simulink model "TiltCopter_TOSTO_v3"  (R2015a)
settings: Solver=ode45  StartTime=0.0  StopTime=10  RelTol=1e-3
values from neighbouring files (symbols this model uses):
  b = 0.55/2    (= 0.275)    [TiltCopter_Parameters_TOSTO_v3.m]
  B0 = 1.399e04    (= 13990)    [TiltCopter_Parameters_TOSTO_v3.m]
  B1 = 1150    [TiltCopter_Parameters_TOSTO_v3.m]
  B2 = 37.46    [TiltCopter_Parameters_TOSTO_v3.m]
  B3 = 1    [TiltCopter_Parameters_TOSTO_v3.m]
  degtorad = pi/180    (= 0.0174532925199)    [TiltCopter_Parameters_TOSTO_v3.m]
  dLMN = [dLdp  0    0 ... (first row only)    [TiltCopter_Parameters_TOSTO_v3.m]
  g = 9.81    [TiltCopter_Parameters_TOSTO_v3.m]
  I_Pi = diag([8.450e-5 8.450e-5 4.580e-5])    [TiltCopter_Parameters_TOSTO_v3.m]
  In = diag([Ixx Iyy Izz])    [TiltCopter_Parameters_TOSTO_v3.m]
  InInv = In\eye(3)    [TiltCopter_Parameters_TOSTO_v3.m]
  KaD = 5.4    [TiltCopter_Parameters_TOSTO_v3.m]
  KaI = 3.6    [TiltCopter_Parameters_TOSTO_v3.m]
  KaN = 38    [TiltCopter_Parameters_TOSTO_v3.m]
  KaP = 8.0    (= 8)    [TiltCopter_Parameters_TOSTO_v3.m]
  Kba = sqrt(KaD/KaI)    [TiltCopter_Parameters_TOSTO_v3.m]
  Kbp = sqrt(Kdp/Kip)    [TiltCopter_Parameters_TOSTO_v3.m]
  Kbq = sqrt(Kdq/Kiq)    [TiltCopter_Parameters_TOSTO_v3.m]
  Kbr = sqrt(Kdr/Kir)    [TiltCopter_Parameters_TOSTO_v3.m]
  Kdp = 0.0499    [TiltCopter_Parameters_TOSTO_v3.m]
  Kdq = 0.0499    [TiltCopter_Parameters_TOSTO_v3.m]
  Kdr = 0.0153    [TiltCopter_Parameters_TOSTO_v3.m]
  Kip = 0.304    [TiltCopter_Parameters_TOSTO_v3.m]
  Kiq = 0.304    [TiltCopter_Parameters_TOSTO_v3.m]
  Kir = 0.125    [TiltCopter_Parameters_TOSTO_v3.m]
  KPD = 0.00512    [TiltCopter_Parameters_TOSTO_v3.m]
  KPP = 1.61    [TiltCopter_Parameters_TOSTO_v3.m]
  Kpp = 0.298    [TiltCopter_Parameters_TOSTO_v3.m]
  Kpq = 0.298    [TiltCopter_Parameters_TOSTO_v3.m]
  Kpr = 0.135    [TiltCopter_Parameters_TOSTO_v3.m]
  Kq = Cq*ro*A*R^3    (= 2.88925724261e-07)    [TiltCopter_Parameters_TOSTO_v3.m]
  KRD = 0.00512    [TiltCopter_Parameters_TOSTO_v3.m]
  KRP = 1.61    [TiltCopter_Parameters_TOSTO_v3.m]
  Kt = Ct*ro*A*R^2    (= 2.46191978476e-05)    [TiltCopter_Parameters_TOSTO_v3.m]
  m = 1.510    (= 1.51)    [TiltCopter_Parameters_TOSTO_v3.m]
  m_servo = p(1)    [TiltCopter_Parameters_TOSTO_v3.m]
  Mb = diag([m m m])    [TiltCopter_Parameters_TOSTO_v3.m]
  MbInv = Mb\eye(3)    [TiltCopter_Parameters_TOSTO_v3.m]
  N = 1/Tf    (= 100)    [TiltCopter_Parameters_TOSTO_v3.m]
  omega_hover = OMEhov    [TiltCopter_Parameters_TOSTO_v3.m]
  pitchMax = pi/6    (= 0.523598775598)    [TiltCopter_Parameters_TOSTO_v3.m]
  q_servo = p(2)    [TiltCopter_Parameters_TOSTO_v3.m]
  rollMax = pi/6    (= 0.523598775598)    [TiltCopter_Parameters_TOSTO_v3.m]
  satp = 1.5    [TiltCopter_Parameters_TOSTO_v3.m]
  satq = 1.5    [TiltCopter_Parameters_TOSTO_v3.m]
  satr = 1    [TiltCopter_Parameters_TOSTO_v3.m]
  ServoMotor_Gain = 1.409e04    (= 14090)    [TiltCopter_Parameters_TOSTO_v3.m]
  tau = 0.055257    [TiltCopter_Parameters_TOSTO_v3.m]
  U = [-1; 0; 0; 0]    [Main_tiltCopter_TOSTO_v3.m]
  x1 = [m q]    [TiltCopter_Parameters_TOSTO_v3.m]
  yawRateMax = pi/2    (= 1.57079632679)    [TiltCopter_Parameters_TOSTO_v3.m]
undefined symbols (not defined in the file or in its folder): i, KPI, KRI
libraries: aerolibutil x10, simulink x6
(part 1 of 2)
settings Model: PauseTimes=2  Creator=Claudio  LastModifiedBy=Claudio

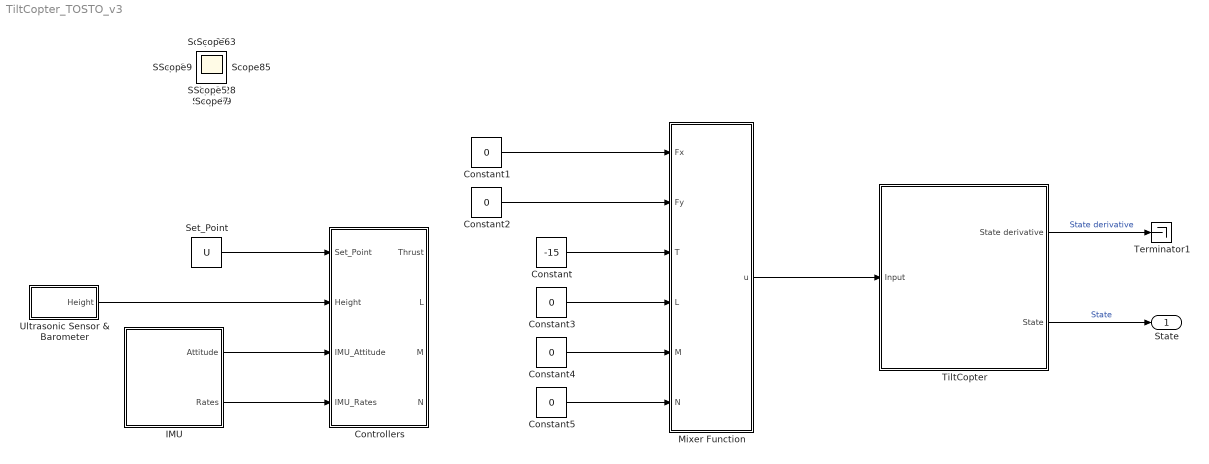
== system TiltCopter_TOSTO_v3 ==
  Constant : Constant  Value=-15
  Constant{1..5} (5 alike) : Constant  Value=0
  Controllers : Subsystem
  IMU : Subsystem
  Mixer Function : Subsystem
  Set_Point : Constant  Value=U
  Terminator1 : Terminator
  TiltCopter : Subsystem
      mask Display:
      | % image(imread(''))
      | port_label('input',1,'u')
      | port_label('output',1,'Xdot')
      | port_label('output',2,'X')
  Ultrasonic Sensor & Barometer : Subsystem
  State : Outport
  Scope{,1..29} (30 alike) : Scope
      Scope settings: SaveName=ScopeData2
      Scope1 settings: SaveName=ScopeData3
      Scope10 settings: SaveName=ScopeData14
      Scope11 settings: SaveName=ScopeData15
      Scope12 settings: SaveName=ScopeData16
      Scope13 settings: SaveName=ScopeData17
      Scope14 settings: SaveName=ScopeData18
      Scope15 settings: SaveName=ScopeData19
      Scope16 settings: SaveName=ScopeData20
      Scope17 settings: SaveName=ScopeData21
      Scope18 settings: SaveName=ScopeData22
      Scope19 settings: SaveName=ScopeData23
      Scope2 settings: SaveName=ScopeData4
      Scope20 settings: SaveName=ScopeData24
      Scope21 settings: SaveName=ScopeData25
      Scope22 settings: SaveName=ScopeData26
      Scope23 settings: SaveName=ScopeData27
      Scope24 settings: SaveName=ScopeData28
      Scope25 settings: SaveName=ScopeData31
      Scope26 settings: SaveName=ScopeData30
      Scope27 settings: ShowLegends=on  SaveName=ScopeData32
      Scope28 settings: SaveName=ScopeData33
      Scope29 settings: SaveName=ScopeData34
      Scope3 settings: SaveName=ScopeData5
      Scope4 settings: SaveName=ScopeData8
      Scope5 settings: TimeRange=20  SaveName=ScopeData9
      Scope6 settings: SaveName=ScopeData10
      Scope7 settings: SaveName=ScopeData11
      Scope8 settings: SaveName=ScopeData12
      Scope9 settings: SaveName=ScopeData13
  wires:
  TiltCopter/2(State) -> State/1  "State"
  TiltCopter/1(State derivative) -> Terminator1/1  "State derivative"
  Constant1/1 -> Mixer Function/1(Fx)
  Constant2/1 -> Mixer Function/2(Fy)
  Mixer Function/1(u) -> TiltCopter/1(Input)
  Set_Point/1 -> Controllers/1(Set_Point)
  IMU/1(Attitude) -> Controllers/3(IMU_Attitude)
  IMU/2(Rates) -> Controllers/4(IMU_Rates)
  Ultrasonic Sensor & Barometer/1(Height) -> Controllers/2(Height)
  Constant/1 -> Mixer Function/3(T)
  Constant5/1 -> Mixer Function/6(N)
  Constant4/1 -> Mixer Function/5(M)
  Constant3/1 -> Mixer Function/4(L)

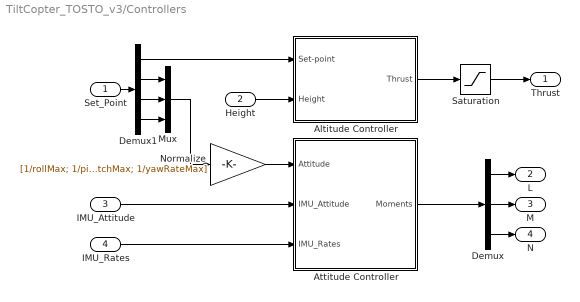
== system TiltCopter_TOSTO_v3/Controllers ==
  Set_Point : Inport
  Height : Inport  Port=2
  IMU_Attitude : Inport  Port=3
  IMU_Rates : Inport  Port=4
  Altitude Controller : Subsystem
  Attitude Controller : Subsystem
  Demux : Demux  Outputs=3
  Demux1 : Demux
  Mux : Mux  Inputs=3
  Normalize : Gain  Gain=[1/rollMax; 1/pitchMax; 1/yawRateMax]
  Saturation : Saturate  UpperLimit=0  LowerLimit=-80
  Thrust : Outport
  L : Outport  Port=2
  M : Outport  Port=3
  N : Outport  Port=4
  wires:
  IMU_Rates/1 -> Attitude Controller/3(IMU_Rates)
  Demux/1 -> L/1
  Demux/2 -> M/1
  Demux/3 -> N/1
  Set_Point/1 -> Demux1/1
  Demux1/3 -> Mux/2
  Demux1/4 -> Mux/3
  IMU_Attitude/1 -> Attitude Controller/2(IMU_Attitude)
  Mux/1 -> Normalize/1
  Normalize/1 -> Attitude Controller/1(Attitude)
  Demux1/1 -> Altitude Controller/1(Set-point)
  Height/1 -> Altitude Controller/2(Height)
  Altitude Controller/1(Thrust) -> Saturation/1
  Saturation/1 -> Thrust/1
  Attitude Controller/1(Moments) -> Demux/1
  Demux1/2 -> Mux/1

== system TiltCopter_TOSTO_v3/IMU ==
  Attitude : Outport
  Rates : Outport  Port=2
  wires:
  [Omega_b] -> Rates/1
  [Alpha_e] -> Attitude/1

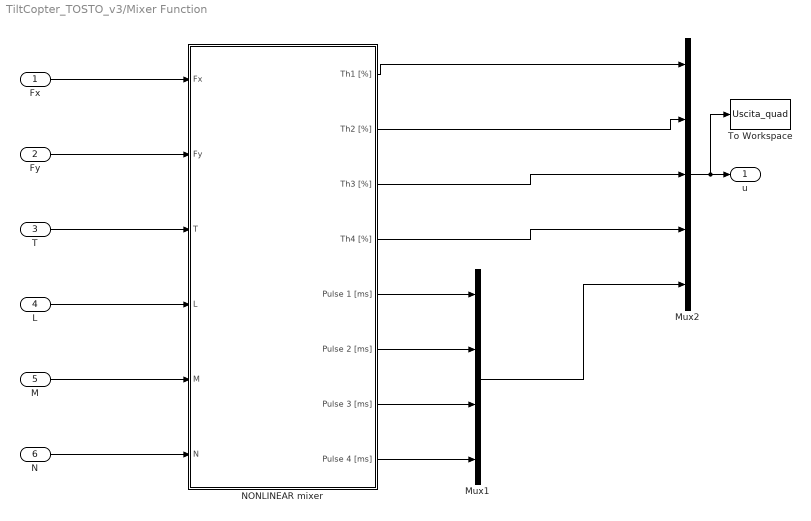
== system TiltCopter_TOSTO_v3/Mixer Function ==
  Fx : Inport
  Fy : Inport  Port=2
  T : Inport  Port=3
  L : Inport  Port=4
  M : Inport  Port=5
  N : Inport  Port=6
  Mux1 : Mux
  Mux2 : Mux  Inputs=5
  NONLINEAR mixer : Subsystem
  To Workspace : ToWorkspace  VariableName=Uscita_quad  SaveFormat=Timeseries  SampleTime=-1
  u : Outport
  wires:
  Mux2/1 -> To Workspace/1, u/1
  Fy/1 -> NONLINEAR mixer/2(Fy)
  Fx/1 -> NONLINEAR mixer/1(Fx)
  T/1 -> NONLINEAR mixer/3(T)
  L/1 -> NONLINEAR mixer/4(L)
  N/1 -> NONLINEAR mixer/6(N)
  M/1 -> NONLINEAR mixer/5(M)
  Mux1/1 -> Mux2/5
  NONLINEAR mixer/5(Pulse 1 [ms]) -> Mux1/1
  NONLINEAR mixer/6(Pulse 2 [ms]) -> Mux1/2
  NONLINEAR mixer/7(Pulse 3 [ms]) -> Mux1/3
  NONLINEAR mixer/8(Pulse 4 [ms]) -> Mux1/4
  NONLINEAR mixer/4(Th4 [%]) -> Mux2/4
  NONLINEAR mixer/3(Th3 [%]) -> Mux2/3
  NONLINEAR mixer/2(Th2 [%]) -> Mux2/2
  NONLINEAR mixer/1(Th1 [%]) -> Mux2/1

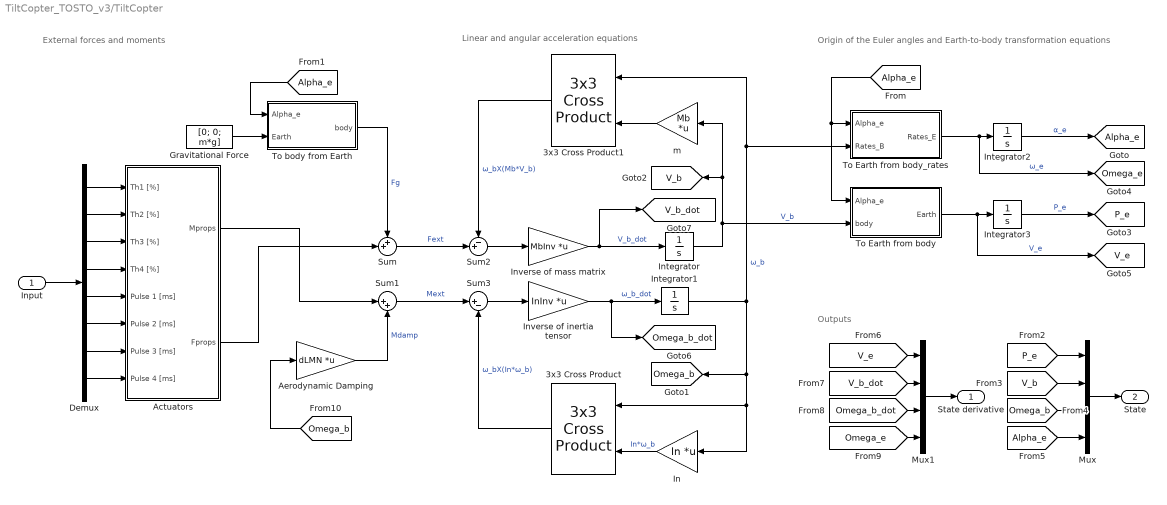
== system TiltCopter_TOSTO_v3/TiltCopter ==
  note: External forces and moments
  note: Outputs
  note: Origin of the Euler angles and Earth-to-body transformation equations
  note: Linear and angular acceleration equations
  Input : Inport
  3x3 Cross Product : aerolibutil/3x3 Cross Product
  3x3 Cross Product1 : aerolibutil/3x3 Cross Product
  Actuators : Subsystem
  Aerodynamic Damping : Gain  Gain=dLMN  Multiplication=Matrix(K*u)
  Demux : Demux  Outputs=8
  Gravitational Force : Constant  Value=[0; 0; m*g]
  In : Gain  Gain=In  Multiplication=Matrix(K*u)
  Integrator : Integrator  InitialCondition=[0; 0; 0]  UpperSaturationLimit=20
  Integrator1 : Integrator  InitialCondition=[0; 0; 0]
  Integrator2 : Integrator  InitialCondition=[0; 0; 0]
  Integrator3 : Integrator  InitialCondition=[0; 0; 0]
  Inverse of inertia tensor : Gain  Gain=InInv  Multiplication=Matrix(K*u)
  Inverse of mass matrix : Gain  Gain=MbInv  Multiplication=Matrix(K*u)
  Mux : Mux
  Mux1 : Mux
  Sum : Sum  Inputs=++|
  Sum1 : Sum  Inputs=|++
  Sum2 : Sum  Inputs=-+|
  Sum3 : Sum  Inputs=|+-
  To Earth from body : MATLAB Function  TreatAsAtomicUnit=on
  To Earth from body_rates : MATLAB Function  TreatAsAtomicUnit=on
  To body from Earth : MATLAB Function  TreatAsAtomicUnit=on
  m : Gain  Gain=Mb  Multiplication=Matrix(K*u)
  State derivative : Outport
  State : Outport  Port=2
  tag scope: Alpha_e=global, Omega_b=global, Omega_b_dot=global, Omega_e=global, P_e=global, V_b=global, V_b_dot=global, V_e=global
  wires:
  To Earth from body_rates/1(Rates_E) -> Integrator2/1, [Omega_e]  "ω_e"
  [P_e] -> Mux/1
  3x3 Cross Product/1 -> Sum3/2  "ω_bX(In*ω_b)"
  [V_b_dot] -> Mux1/2
  Mux/1 -> State/1
  Mux1/1 -> State derivative/1
  [V_b] -> Mux/2
  [Alpha_e] -> Mux/4
  [Omega_b] -> Mux/3
  Demux/4 -> Actuators/4(Th4 [%])
  [Omega_e] -> Mux1/4
  [Omega_b_dot] -> Mux1/3
  [V_e] -> Mux1/1
  Demux/3 -> Actuators/3(Th3 [%])
  Inverse of mass matrix/1 -> Integrator/1, [V_b_dot]  "V_b_dot"
  Integrator/1 -> To Earth from body/2(body), m/1, [V_b]  "V_b"
  [Alpha_e] -> To Earth from body/1(Alpha_e), To Earth from body_rates/1(Alpha_e)
  Integrator1/1 -> To Earth from body_rates/2(Rates_B), 3x3 Cross Product1/1, 3x3 Cross Product/1, In/1, [Omega_b]  "ω_b"
  Sum3/1 -> Inverse of inertia tensor/1
  Sum2/1 -> Inverse of mass matrix/1
  m/1 -> 3x3 Cross Product1/2
  Sum/1 -> Sum2/2  "Fext"
  Sum1/1 -> Sum3/1  "Mext"
  Demux/1 -> Actuators/1(Th1 [%])
  Demux/2 -> Actuators/2(Th2 [%])
  Inverse of inertia tensor/1 -> Integrator1/1, [Omega_b_dot]  "ω_b_dot"
  3x3 Cross Product1/1 -> Sum2/1  "ω_bX(Mb*V_b)"
  Integrator2/1 -> [Alpha_e]  "α_e"
  Aerodynamic Damping/1 -> Sum1/2  "Mdamp"
  Integrator3/1 -> [P_e]  "P_e"
  In/1 -> 3x3 Cross Product/2  "In*ω_b"
  [Omega_b] -> Aerodynamic Damping/1
  To Earth from body/1(Earth) -> [V_e], Integrator3/1  "V_e"
  To body from Earth/1(body) -> Sum/1  "Fg"
  Gravitational Force/1 -> To body from Earth/2(Earth)
  [Alpha_e] -> To body from Earth/1(Alpha_e)
  Input/1 -> Demux/1
  Demux/5 -> Actuators/5(Pulse 1 [ms])
  Demux/6 -> Actuators/6(Pulse 2 [ms])
  Demux/7 -> Actuators/7(Pulse 3 [ms])
  Demux/8 -> Actuators/8(Pulse 4 [ms])
  Actuators/1(Mprops) -> Sum1/1
  Actuators/2(Fprops) -> Sum/2

== system TiltCopter_TOSTO_v3/Ultrasonic Sensor & Barometer ==
  Bias_u : Bias
  Demux : Demux  Outputs=3
  Sum : Sum  Inputs=|++
  Terminator1 : Terminator
  Terminator2 : Terminator
  White Noise_u : RandomNumber  DisableCoverage=on  Variance=0*0.00001  SampleTime=0.01
  Height : Outport
  wires:
  Sum/1 -> Height/1
  Demux/2 -> Terminator1/1  "E"
  [P_e] -> Demux/1
  Bias_u/1 -> Sum/1
  White Noise_u/1 -> Sum/2
  Demux/3 -> Bias_u/1  "D"
  Demux/1 -> Terminator2/1  "N"

== system TiltCopter_TOSTO_v3/Controllers/Altitude Controller ==
  Set-point : Inport
  Height : Inport  Port=2
  Constant : Constant  Value=m*g
  Normalize : Gain
  PD Controller : simulink/Continuous/PID Controller  Controller=PID  TimeDomain=Continuous-time  SampleTime=-1  IntegratorMethod=Forward Euler  FilterMethod=Trapezoidal  Form=Parallel  UseFilter=on  ControllerParametersSource=internal  P=KaP  I=KaI  D=KaD  N=KaN  InitialConditionSource=internal  InitialConditionForIntegrator=0  InitialConditionForFilter=0  ExternalReset=none  LimitOutput=on  UpperSaturationLimit=10  LowerSaturationLimit=-10  LinearizeAsGain=on  AntiWindupMode=back-calculation  Kb=Kba  TrackingMode=off  Kt=1  PParamMin=[]  PParamMax=[]  IParamMin=[]  IParamMax=[]  DParamMin=[]  DParamMax=[]  NParamMin=[]  NParamMax=[]  KbParamMin=[]  KbParamMax=[]  KtParamMin=[]  KtParamMax=[]  POutMin=[]  POutMax=[]  IOutMin=[]  IOutMax=[]  DOutMin=[]  DOutMax=[]  NOutMin=[]  NOutMax=[]  KbOutMin=[]  KbOutMax=[]  KtOutMin=[]  KtOutMax=[]  IntegratorOutMin=[]  IntegratorOutMax=[]  FilterOutMin=[]  FilterOutMax=[]  SumOutMin=[]  SumOutMax=[]  SumI1OutMin=[]  SumI1OutMax=[]  SumI2OutMin=[]  SumI2OutMax=[]  SumI3OutMin=[]  SumI3OutMax=[]  SumDOutMin=[]  SumDOutMax=[]  SaturationOutMin=[]  SaturationOutMax=[]  IntegratorContinuousStateAttributes=''  IntegratorStateMustResolveToSignalObject=off  IntegratorRTWStateStorageClass=Auto  FilterContinuousStateAttributes=''  FilterStateMustResolveToSignalObject=off  FilterRTWStateStorageClass=Auto  DifferentiatorICPrevScaledInput=0  DifferentiatorOutMin=[]  DifferentiatorOutMax=[]
  Sum1 : Sum  Inputs=-+|
  Sum2 : Sum  Inputs=|+-
  Thrust : Outport
  wires:
  Sum2/1 -> PD Controller/1
  Height/1 -> Sum2/2
  Sum1/1 -> Thrust/1
  Constant/1 -> Sum1/1
  Set-point/1 -> Sum2/1
  PD Controller/1 -> Normalize/1
  Normalize/1 -> Sum1/2

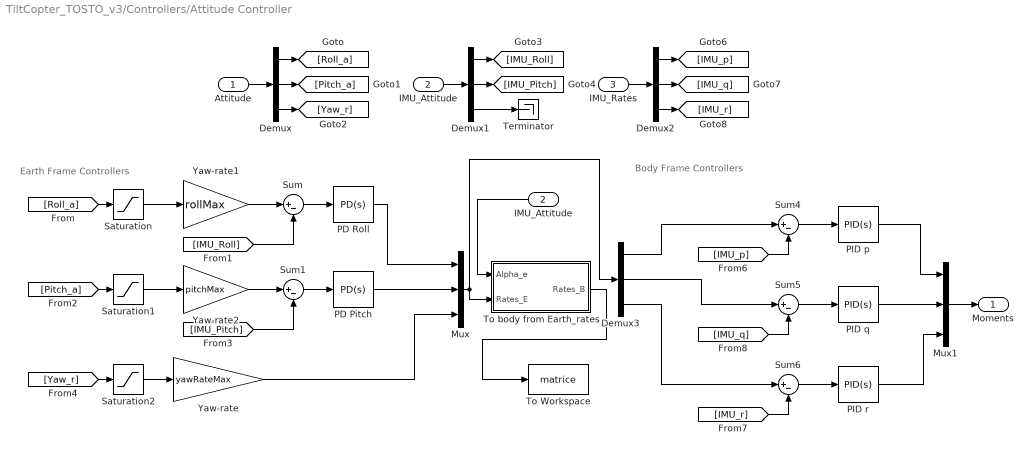
== system TiltCopter_TOSTO_v3/Controllers/Attitude Controller ==
  note: Body Frame Controllers
  note: Earth Frame Controllers
  Attitude : Inport
  IMU_Attitude : Inport  Port=2
  IMU_Rates : Inport  Port=3
  Demux{,1..3} (4 alike) : Demux  Outputs=3
  "IMU_Attitude " : InportShadow  Port=2
  Mux : Mux  Inputs=3
  Mux1 : Mux  Inputs=3
  PD Pitch : simulink/Continuous/PID Controller  Controller=PD  TimeDomain=Continuous-time  SampleTime=-1  IntegratorMethod=Forward Euler  FilterMethod=Forward Euler  Form=Parallel  UseFilter=on  ControllerParametersSource=internal  P=KPP  I=KPI  D=KPD  N=N  InitialConditionSource=internal  InitialConditionForIntegrator=0  InitialConditionForFilter=0  ExternalReset=none  LimitOutput=off  UpperSaturationLimit=inf  LowerSaturationLimit=-inf  LinearizeAsGain=on  AntiWindupMode=none  Kb=1  TrackingMode=off  Kt=1  PParamMin=[]  PParamMax=[]  IParamMin=[]  IParamMax=[]  DParamMin=[]  DParamMax=[]  NParamMin=[]  NParamMax=[]  KbParamMin=[]  KbParamMax=[]  KtParamMin=[]  KtParamMax=[]  POutMin=[]  POutMax=[]  IOutMin=[]  IOutMax=[]  DOutMin=[]  DOutMax=[]  NOutMin=[]  NOutMax=[]  KbOutMin=[]  KbOutMax=[]  KtOutMin=[]  KtOutMax=[]  IntegratorOutMin=[]  IntegratorOutMax=[]  FilterOutMin=[]  FilterOutMax=[]  SumOutMin=[]  SumOutMax=[]  SumI1OutMin=[]  SumI1OutMax=[]  SumI2OutMin=[]  SumI2OutMax=[]  SumI3OutMin=[]  SumI3OutMax=[]  SumDOutMin=[]  SumDOutMax=[]  SaturationOutMin=[]  SaturationOutMax=[]  IntegratorContinuousStateAttributes=''  IntegratorStateMustResolveToSignalObject=off  IntegratorRTWStateStorageClass=Auto  FilterContinuousStateAttributes=''  FilterStateMustResolveToSignalObject=off  FilterRTWStateStorageClass=Auto  DifferentiatorICPrevScaledInput=0  DifferentiatorOutMin=[]  DifferentiatorOutMax=[]
  PD Roll : simulink/Continuous/PID Controller  Controller=PD  TimeDomain=Continuous-time  SampleTime=-1  IntegratorMethod=Forward Euler  FilterMethod=Forward Euler  Form=Parallel  UseFilter=on  ControllerParametersSource=internal  P=KRP  I=KRI  D=KRD  N=N  InitialConditionSource=internal  InitialConditionForIntegrator=0  InitialConditionForFilter=0  ExternalReset=none  LimitOutput=off  UpperSaturationLimit=inf  LowerSaturationLimit=-inf  LinearizeAsGain=on  AntiWindupMode=none  Kb=1  TrackingMode=off  Kt=1  PParamMin=[]  PParamMax=[]  IParamMin=[]  IParamMax=[]  DParamMin=[]  DParamMax=[]  NParamMin=[]  NParamMax=[]  KbParamMin=[]  KbParamMax=[]  KtParamMin=[]  KtParamMax=[]  POutMin=[]  POutMax=[]  IOutMin=[]  IOutMax=[]  DOutMin=[]  DOutMax=[]  NOutMin=[]  NOutMax=[]  KbOutMin=[]  KbOutMax=[]  KtOutMin=[]  KtOutMax=[]  IntegratorOutMin=[]  IntegratorOutMax=[]  FilterOutMin=[]  FilterOutMax=[]  SumOutMin=[]  SumOutMax=[]  SumI1OutMin=[]  SumI1OutMax=[]  SumI2OutMin=[]  SumI2OutMax=[]  SumI3OutMin=[]  SumI3OutMax=[]  SumDOutMin=[]  SumDOutMax=[]  SaturationOutMin=[]  SaturationOutMax=[]  IntegratorContinuousStateAttributes=''  IntegratorStateMustResolveToSignalObject=off  IntegratorRTWStateStorageClass=Auto  FilterContinuousStateAttributes=''  FilterStateMustResolveToSignalObject=off  FilterRTWStateStorageClass=Auto  DifferentiatorICPrevScaledInput=0  DifferentiatorOutMin=[]  DifferentiatorOutMax=[]
  PID p : simulink/Continuous/PID Controller  Controller=PID  TimeDomain=Continuous-time  SampleTime=-1  IntegratorMethod=Forward Euler  FilterMethod=Forward Euler  Form=Parallel  UseFilter=on  ControllerParametersSource=internal  P=Kpp  I=Kip  D=Kdp  N=N  InitialConditionSource=internal  InitialConditionForIntegrator=0  InitialConditionForFilter=0  ExternalReset=none  LimitOutput=on  UpperSaturationLimit=satp  LowerSaturationLimit=-satp  LinearizeAsGain=on  AntiWindupMode=back-calculation  Kb=Kbp  TrackingMode=off  Kt=1  PParamMin=[]  PParamMax=[]  IParamMin=[]  IParamMax=[]  DParamMin=[]  DParamMax=[]  NParamMin=[]  NParamMax=[]  KbParamMin=[]  KbParamMax=[]  KtParamMin=[]  KtParamMax=[]  POutMin=[]  POutMax=[]  IOutMin=[]  IOutMax=[]  DOutMin=[]  DOutMax=[]  NOutMin=[]  NOutMax=[]  KbOutMin=[]  KbOutMax=[]  KtOutMin=[]  KtOutMax=[]  IntegratorOutMin=[]  IntegratorOutMax=[]  FilterOutMin=[]  FilterOutMax=[]  SumOutMin=[]  SumOutMax=[]  SumI1OutMin=[]  SumI1OutMax=[]  SumI2OutMin=[]  SumI2OutMax=[]  SumI3OutMin=[]  SumI3OutMax=[]  SumDOutMin=[]  SumDOutMax=[]  SaturationOutMin=[]  SaturationOutMax=[]  IntegratorContinuousStateAttributes=''  IntegratorStateMustResolveToSignalObject=off  IntegratorRTWStateStorageClass=Auto  FilterContinuousStateAttributes=''  FilterStateMustResolveToSignalObject=off  FilterRTWStateStorageClass=Auto  DifferentiatorICPrevScaledInput=0  DifferentiatorOutMin=[]  DifferentiatorOutMax=[]
  PID q : simulink/Continuous/PID Controller  Controller=PID  TimeDomain=Continuous-time  SampleTime=-1  IntegratorMethod=Forward Euler  FilterMethod=Forward Euler  Form=Parallel  UseFilter=on  ControllerParametersSource=internal  P=Kpq  I=Kiq  D=Kdq  N=N  InitialConditionSource=internal  InitialConditionForIntegrator=0  InitialConditionForFilter=0  ExternalReset=none  LimitOutput=on  UpperSaturationLimit=satq  LowerSaturationLimit=-satq  LinearizeAsGain=on  AntiWindupMode=back-calculation  Kb=Kbq  TrackingMode=off  Kt=1  PParamMin=[]  PParamMax=[]  IParamMin=[]  IParamMax=[]  DParamMin=[]  DParamMax=[]  NParamMin=[]  NParamMax=[]  KbParamMin=[]  KbParamMax=[]  KtParamMin=[]  KtParamMax=[]  POutMin=[]  POutMax=[]  IOutMin=[]  IOutMax=[]  DOutMin=[]  DOutMax=[]  NOutMin=[]  NOutMax=[]  KbOutMin=[]  KbOutMax=[]  KtOutMin=[]  KtOutMax=[]  IntegratorOutMin=[]  IntegratorOutMax=[]  FilterOutMin=[]  FilterOutMax=[]  SumOutMin=[]  SumOutMax=[]  SumI1OutMin=[]  SumI1OutMax=[]  SumI2OutMin=[]  SumI2OutMax=[]  SumI3OutMin=[]  SumI3OutMax=[]  SumDOutMin=[]  SumDOutMax=[]  SaturationOutMin=[]  SaturationOutMax=[]  IntegratorContinuousStateAttributes=''  IntegratorStateMustResolveToSignalObject=off  IntegratorRTWStateStorageClass=Auto  FilterContinuousStateAttributes=''  FilterStateMustResolveToSignalObject=off  FilterRTWStateStorageClass=Auto  DifferentiatorICPrevScaledInput=0  DifferentiatorOutMin=[]  DifferentiatorOutMax=[]
  PID r : simulink/Continuous/PID Controller  Controller=PID  TimeDomain=Continuous-time  SampleTime=-1  IntegratorMethod=Forward Euler  FilterMethod=Forward Euler  Form=Parallel  UseFilter=on  ControllerParametersSource=internal  P=Kpr  I=Kir  D=Kdr  N=N  InitialConditionSource=internal  InitialConditionForIntegrator=0  InitialConditionForFilter=0  ExternalReset=none  LimitOutput=on  UpperSaturationLimit=satr  LowerSaturationLimit=-satr  LinearizeAsGain=on  AntiWindupMode=back-calculation  Kb=Kbr  TrackingMode=off  Kt=1  PParamMin=[]  PParamMax=[]  IParamMin=[]  IParamMax=[]  DParamMin=[]  DParamMax=[]  NParamMin=[]  NParamMax=[]  KbParamMin=[]  KbParamMax=[]  KtParamMin=[]  KtParamMax=[]  POutMin=[]  POutMax=[]  IOutMin=[]  IOutMax=[]  DOutMin=[]  DOutMax=[]  NOutMin=[]  NOutMax=[]  KbOutMin=[]  KbOutMax=[]  KtOutMin=[]  KtOutMax=[]  IntegratorOutMin=[]  IntegratorOutMax=[]  FilterOutMin=[]  FilterOutMax=[]  SumOutMin=[]  SumOutMax=[]  SumI1OutMin=[]  SumI1OutMax=[]  SumI2OutMin=[]  SumI2OutMax=[]  SumI3OutMin=[]  SumI3OutMax=[]  SumDOutMin=[]  SumDOutMax=[]  SaturationOutMin=[]  SaturationOutMax=[]  IntegratorContinuousStateAttributes=''  IntegratorStateMustResolveToSignalObject=off  IntegratorRTWStateStorageClass=Auto  FilterContinuousStateAttributes=''  FilterStateMustResolveToSignalObject=off  FilterRTWStateStorageClass=Auto  DifferentiatorICPrevScaledInput=0  DifferentiatorOutMin=[]  DifferentiatorOutMax=[]
  Saturation : Saturate  UpperLimit=1  LowerLimit=-1
  Saturation1 : Saturate  UpperLimit=1  LowerLimit=-1
  Saturation2 : Saturate  UpperLimit=1  LowerLimit=-1
  Sum{,1,4..6} (5 alike) : Sum  Inputs=|+-
  Terminator : Terminator
  To Workspace : ToWorkspace  VariableName=matrice  SaveFormat=Timeseries  SampleTime=-1
  To body from Earth_rates : MATLAB Function  TreatAsAtomicUnit=on
  Yaw-rate : Gain  Gain=yawRateMax
  Yaw-rate1 : Gain  Gain=rollMax
  Yaw-rate2 : Gain  Gain=pitchMax
  Moments : Outport
  wires:
  Sum4/1 -> PID p/1
  IMU_Attitude/1 -> Demux1/1
  Attitude/1 -> Demux/1
  Demux/3 -> [Yaw_r]
  IMU_Rates/1 -> Demux2/1
  [IMU_Pitch] -> Sum1/2
  [Pitch_a] -> Saturation1/1
  [IMU_Roll] -> Sum/2
  [Roll_a] -> Saturation/1
  Mux1/1 -> Moments/1
  PD Roll/1 -> Mux/1
  [Yaw_r] -> Saturation2/1
  PD Pitch/1 -> Mux/2
  Sum5/1 -> PID q/1
  PID r/1 -> Mux1/3
  PID p/1 -> Mux1/1
  Sum6/1 -> PID r/1
  PID q/1 -> Mux1/2
  Demux/2 -> [Pitch_a]
  Demux2/3 -> [IMU_r]
  Demux1/1 -> [IMU_Roll]
  Demux/1 -> [Roll_a]
  Demux2/1 -> [IMU_p]
  Demux1/3 -> Terminator/1
  Demux2/2 -> [IMU_q]
  Demux1/2 -> [IMU_Pitch]
  Sum/1 -> PD Roll/1
  Sum1/1 -> PD Pitch/1
  Saturation1/1 -> Yaw-rate2/1
  Yaw-rate1/1 -> Sum/1
  Yaw-rate2/1 -> Sum1/1
  Demux3/1 -> Sum4/1
  [IMU_p] -> Sum4/2
  Demux3/2 -> Sum5/1
  Demux3/3 -> Sum6/1
  [IMU_q] -> Sum5/2
  [IMU_r] -> Sum6/2
  Yaw-rate/1 -> Mux/3
  Saturation/1 -> Yaw-rate1/1
  Saturation2/1 -> Yaw-rate/1
  "IMU_Attitude "/1 -> To body from Earth_rates/1(Alpha_e)
  To body from Earth_rates/1(Rates_B) -> To Workspace/1
  Mux/1 -> Demux3/1, To body from Earth_rates/2(Rates_E)

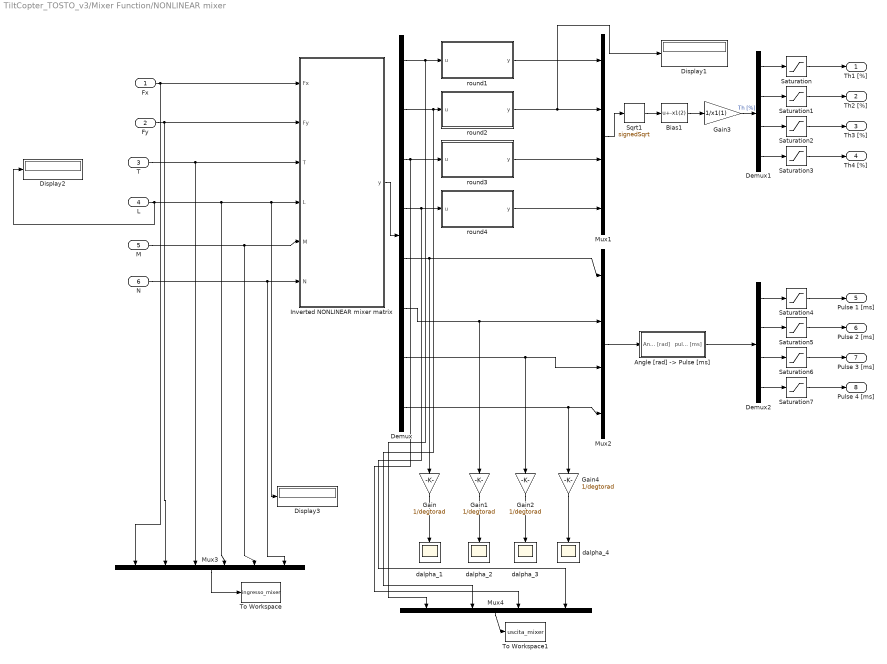
== system TiltCopter_TOSTO_v3/Mixer Function/NONLINEAR mixer ==
  Fx : Inport
  Fy : Inport  Port=2
  T : Inport  Port=3
  L : Inport  Port=4
  M : Inport  Port=5
  N : Inport  Port=6
  "Angle [rad] -> Pulse [ms]" : Subsystem
  Bias1 : Bias  Bias=-x1(2)
  Demux : Demux  Outputs=8
  Demux1 : Demux
  Demux2 : Demux
  Display1 : Display
  Display2 : Display
  Display3 : Display
  Gain{,1..2,4} (4 alike) : Gain  Gain=1/degtorad
  Gain3 : Gain  Gain=1/x1(1)
  Inverted NONLINEAR mixer matrix : MATLAB Function  TreatAsAtomicUnit=on
  Mux1 : Mux
  Mux2 : Mux
  Mux3 : Mux  Inputs=6
  Mux4 : Mux
  Saturation{,1..3} (4 alike) : Saturate  UpperLimit=100  LowerLimit=0
  Saturation{4..7} (4 alike) : Saturate  UpperLimit=2000  LowerLimit=1000
  Sqrt1 : Sqrt  Operator=signedSqrt  SaturateOnIntegerOverflow=on
  To Workspace : ToWorkspace  VariableName=ingresso_mixer  SaveFormat=Structure With Time  SampleTime=-1
  To Workspace1 : ToWorkspace  VariableName=uscita_mixer  SaveFormat=Structure With Time  SampleTime=-1
  dalpha_{1..4} (4 alike) : Scope
      dalpha_3 settings: SaveName=ScopeData6
      dalpha_4 settings: SaveName=ScopeData7
  round1 : MATLAB Function  TreatAsAtomicUnit=on
  round2 : MATLAB Function  TreatAsAtomicUnit=on
  round3 : MATLAB Function  TreatAsAtomicUnit=on
  round4 : MATLAB Function  TreatAsAtomicUnit=on
  Th1 [%] : Outport
  Th2 [%] : Outport  Port=2
  Th3 [%] : Outport  Port=3
  Th4 [%] : Outport  Port=4
  Pulse 1 [ms] : Outport  Port=5
  Pulse 2 [ms] : Outport  Port=6
  Pulse 3 [ms] : Outport  Port=7
  Pulse 4 [ms] : Outport  Port=8
  wires:
  round1/1(y) -> Mux1/1
  Saturation6/1 -> Pulse 3 [ms]/1
  Demux2/1 -> Saturation4/1
  Demux2/3 -> Saturation6/1
  Demux/4 -> Mux4/4, round4/1(u)
  Saturation2/1 -> Th3 [%]/1
  Demux1/2 -> Saturation1/1
  Demux1/1 -> Saturation/1
  Demux1/3 -> Saturation2/1
  Demux1/4 -> Saturation3/1
  Saturation1/1 -> Th2 [%]/1
  Gain3/1 -> Demux1/1  "Th [%]"
  Sqrt1/1 -> Bias1/1
  Mux1/1 -> Sqrt1/1
  Demux/1 -> Mux4/1, round1/1(u)
  Bias1/1 -> Gain3/1
  Saturation3/1 -> Th4 [%]/1
  Saturation/1 -> Th1 [%]/1
  Demux2/2 -> Saturation5/1
  round2/1(y) -> Display1/1, Mux1/2
  round4/1(y) -> Mux1/4
  Demux/7 -> Gain2/1, Mux2/3
  Demux/5 -> Gain/1, Mux2/1
  Demux/6 -> Mux2/2, Gain1/1
  Mux2/1 -> "Angle [rad] -> Pulse [ms]"/1(Angle [rad])
  Demux2/4 -> Saturation7/1
  Demux/3 -> round3/1(u), Mux4/3
  Demux/8 -> Mux2/4, Gain4/1
  "Angle [rad] -> Pulse [ms]"/1(pulse [ms]) -> Demux2/1
  Saturation4/1 -> Pulse 1 [ms]/1
  Saturation5/1 -> Pulse 2 [ms]/1
  Saturation7/1 -> Pulse 4 [ms]/1
  Gain1/1 -> dalpha_2/1
  Gain/1 -> dalpha_1/1
  Gain2/1 -> dalpha_3/1
  Gain4/1 -> dalpha_4/1
  round3/1(y) -> Mux1/3
  Inverted NONLINEAR mixer matrix/1(y) -> Demux/1
  Demux/2 -> Mux4/2, round2/1(u)
  Fx/1 -> Mux3/1, Inverted NONLINEAR mixer matrix/1(Fx)
  Fy/1 -> Inverted NONLINEAR mixer matrix/2(Fy), Mux3/2
  T/1 -> Inverted NONLINEAR mixer matrix/3(T), Mux3/3
  L/1 -> Mux3/4, Display3/1, Inverted NONLINEAR mixer matrix/4(L), Display2/1
  M/1 -> Mux3/5, Inverted NONLINEAR mixer matrix/5(M)
  N/1 -> Mux3/6, Inverted NONLINEAR mixer matrix/6(N)
  Mux3/1 -> To Workspace/1
  Mux4/1 -> To Workspace1/1

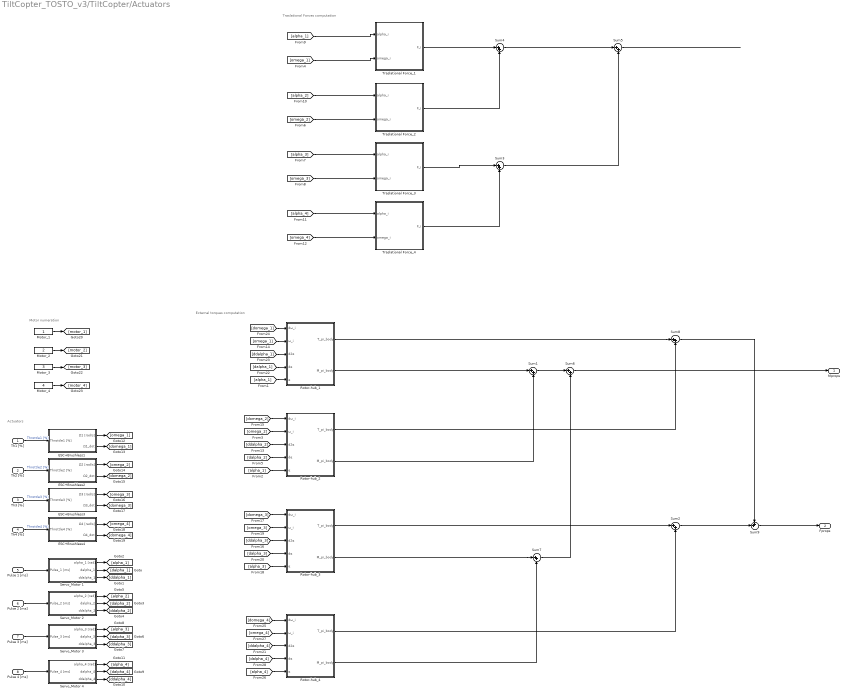
== system TiltCopter_TOSTO_v3/TiltCopter/Actuators ==
  note: Actuators
  note: Motor numeration
  note: Traslational Forces computation
  note: External torques computation
  Th1 [%] : Inport
  Th2 [%] : Inport  Port=2
  Th3 [%] : Inport  Port=3
  Th4 [%] : Inport  Port=4
  Pulse 1 [ms] : Inport  Port=5
  Pulse 2 [ms] : Inport  Port=6
  Pulse 3 [ms] : Inport  Port=7
  Pulse 4 [ms] : Inport  Port=8
  ESC+Brushless1 : Subsystem
  ESC+Brushless2 : Subsystem
  ESC+Brushless3 : Subsystem
  ESC+Brushless4 : Subsystem
  Motor_1 : Constant
  Motor_2 : Constant  Value=2
  Motor_3 : Constant  Value=3
  Motor_4 : Constant  Value=4
  Rotor-hub_1 : Subsystem
  Rotor-hub_2 : Subsystem
  Rotor-hub_3 : Subsystem
  Rotor-hub_4 : Subsystem
  Servo_Motor 1 : Subsystem
  Servo_Motor 2 : Subsystem
  Servo_Motor 3 : Subsystem
  Servo_Motor 4 : Subsystem
  Sum{1..8} (8 alike) : Sum  Inputs=|++
  Sum9 : Sum  Inputs=++|
  Traslational Force_1 : Subsystem
  Traslational Force_2 : Subsystem
  Traslational Force_3 : Subsystem
  Traslational Force_4 : Subsystem
  Mprops : Outport
  Fprops : Outport  Port=2
  wires:
  Th1 [%]/1 -> ESC+Brushless1/1(Throttle1 [%])  "Throttle1 [%]"
  Th2 [%]/1 -> ESC+Brushless2/1(Throttle2 [%])  "Throttle2 [%]"
  Th4 [%]/1 -> ESC+Brushless4/1(Throttle4 [%])  "Throttle4 [%]"
  Th3 [%]/1 -> ESC+Brushless3/1(Throttle3 [%])  "Throttle3 [%]"
  Pulse 1 [ms]/1 -> Servo_Motor 1/1(Pulse_1 [ms])
  Pulse 2 [ms]/1 -> Servo_Motor 2/1(Pulse_2 [ms])
  Pulse 3 [ms]/1 -> Servo_Motor 3/1(Pulse_3 [ms])
  Pulse 4 [ms]/1 -> Servo_Motor 4/1(Pulse_4 [ms])
  Servo_Motor 1/2(dalpha_1) -> [dalpha_1]
  Servo_Motor 1/3(ddalpha_1) -> [ddalpha_1]
  Servo_Motor 3/1(alpha_3 [rad]) -> [alpha_3]
  Servo_Motor 3/3(ddalpha_3) -> [ddalpha_3]
  Servo_Motor 3/2(dalpha_3) -> [dalpha_3]
  Servo_Motor 2/3(ddalpha_2) -> [ddalpha_2]
  Servo_Motor 2/2(dalpha_2) -> [dalpha_2]
  Servo_Motor 2/1(alpha_2 [rad]) -> [alpha_2]
  Servo_Motor 1/1(alpha_1 [rad]) -> [alpha_1]
  Servo_Motor 4/1(alpha_4 [rad]) -> [alpha_4]
  Servo_Motor 4/2(dalpha_4) -> [dalpha_4]
  Servo_Motor 4/3(ddalpha_4) -> [ddalpha_4]
  ESC+Brushless1/1(Ω1 [rad/s]) -> [omega_1]
  ESC+Brushless1/2(Ω1_dot) -> [domega_1]
  ESC+Brushless2/1(Ω2 [rad/s]) -> [omega_2]
  ESC+Brushless2/2(Ω2_dot) -> [domega_2]
  ESC+Brushless3/1(Ω3 [rad/s]) -> [omega_3]
  ESC+Brushless3/2(Ω3_dot) -> [domega_3]
  ESC+Brushless4/1(Ω4 [rad/s]) -> [omega_4]
  ESC+Brushless4/2("Ω4_dot ") -> [domega_4]
  [omega_2] -> Traslational Force_2/2(omega_i)
  [alpha_1] -> Traslational Force_1/1(alpha_i)
  [omega_1] -> Traslational Force_1/2(omega_i)
  [alpha_2] -> Traslational Force_2/1(alpha_i)
  Motor_1/1 -> [motor_1]
  Motor_2/1 -> [motor_2]
  Motor_3/1 -> [motor_3]
  Motor_4/1 -> [motor_4]
  [omega_3] -> Traslational Force_3/2(omega_i)
  [alpha_3] -> Traslational Force_3/1(alpha_i)
  [omega_4] -> Traslational Force_4/2(omega_i)
  [alpha_4] -> Traslational Force_4/1(alpha_i)
  Traslational Force_3/1(F_i) -> Sum3/1
  Traslational Force_4/1(F_i) -> Sum3/2
  Traslational Force_1/1(F_i) -> Sum4/1
  Traslational Force_2/1(F_i) -> Sum4/2
  Sum4/1 -> Sum5/1
  Sum3/1 -> Sum5/2
  Sum5/1 -> ?
  [ddalpha_1] -> Rotor-hub_1/3(d2α)
  [dalpha_1] -> Rotor-hub_1/4(dα)
  [alpha_1] -> Rotor-hub_1/5(α)
  [domega_1] -> Rotor-hub_1/1(dω_i)
  [omega_1] -> Rotor-hub_1/2(ω_i)
  [domega_2] -> Rotor-hub_2/1(dω_i)
  [omega_2] -> Rotor-hub_2/2(ω_i)
  [ddalpha_2] -> Rotor-hub_2/3(d2α)
  [dalpha_2] -> Rotor-hub_2/4(dα)
  [alpha_1] -> Rotor-hub_2/5(α)
  [domega_3] -> Rotor-hub_3/1(dω_i)
  [omega_3] -> Rotor-hub_3/2(ω_i)
  [ddalpha_3] -> Rotor-hub_3/3(d2α)
  [dalpha_3] -> Rotor-hub_3/4(dα)
  [alpha_3] -> Rotor-hub_3/5(α)
  [domega_4] -> Rotor-hub_4/1(dω_i)
  [omega_4] -> Rotor-hub_4/2(ω_i)
  [ddalpha_4] -> Rotor-hub_4/3(d2α)
  [dalpha_4] -> Rotor-hub_4/4(dα)
  [alpha_4] -> Rotor-hub_4/5(α)
  Rotor-hub_1/2(" M_pi_body") -> Sum1/1
  Rotor-hub_2/2(" M_pi_body") -> Sum1/2
  Sum1/1 -> Sum6/1
  Rotor-hub_3/2(" M_pi_body") -> Sum7/1
  Rotor-hub_4/2(" M_pi_body") -> Sum7/2
  Sum7/1 -> Sum6/2
  Sum6/1 -> Mprops/1
  Rotor-hub_3/1(" T_pi_body") -> Sum2/1
  Rotor-hub_4/1(" T_pi_body") -> Sum2/2
  Rotor-hub_1/1(" T_pi_body") -> Sum8/1
  Rotor-hub_2/1(" T_pi_body") -> Sum8/2
  Sum8/1 -> Sum9/1
  Sum2/1 -> Sum9/2
  Sum9/1 -> Fprops/1

== system TiltCopter_TOSTO_v3/Mixer Function/NONLINEAR mixer/Angle [rad] -> Pulse [ms] ==
  Angle [rad] : Inport
  Add : Sum
  Constant : Constant  Value=q_servo
  Linear fitting gain : Gain  Gain=m_servo
  pulse [ms] : Outport
  wires:
  Angle [rad]/1 -> Linear fitting gain/1
  Constant/1 -> Add/2
  Linear fitting gain/1 -> Add/1
  Add/1 -> pulse [ms]/1

== system TiltCopter_TOSTO_v3/TiltCopter/Actuators/ESC+Brushless1 ==
  note: questo blocco è stato introdotto per avere in
      | uscita l'accelerazione e la velocità
  Throttle1 [%] : Inport
  Bias : Bias  Bias=x1(2)
  Gain : Gain  Gain=x1(1)
  Integrator : Integrator
  Transfer Fcn : TransferFcn  Numerator=[-1 0]  Denominator=[(tau) 1]
  Ω1 [rad/s] : Outport
  Ω1_dot : Outport  Port=2
  wires:
  Gain/1 -> Transfer Fcn/1
  Throttle1 [%]/1 -> Gain/1
  Transfer Fcn/1 -> Ω1_dot/1, Integrator/1
  Integrator/1 -> Bias/1
  Bias/1 -> Ω1 [rad/s]/1

== system TiltCopter_TOSTO_v3/TiltCopter/Actuators/ESC+Brushless2 ==
  Throttle2 [%] : Inport
  Bias : Bias  Bias=x1(2)
  Derivative : Derivative
  Gain : Gain  Gain=x1(1)
  Integrator : Integrator
  Transfer Fcn : TransferFcn  Numerator=[-1 0]  Denominator=[(tau) 1]
  Ω2 [rad/s] : Outport
  Ω2_dot : Outport  Port=2
  wires:
  Derivative/1 -> Ω2_dot/1
  Gain/1 -> Transfer Fcn/1
  Throttle2 [%]/1 -> Gain/1
  Transfer Fcn/1 -> Derivative/1, Integrator/1
  Integrator/1 -> Bias/1
  Bias/1 -> Ω2 [rad/s]/1

== system TiltCopter_TOSTO_v3/TiltCopter/Actuators/ESC+Brushless3 ==
  Throttle3 [%] : Inport
  Bias : Bias  Bias=x1(2)
  Gain : Gain  Gain=x1(1)
  Integrator : Integrator
  Transfer Fcn : TransferFcn  Numerator=[-1 0]  Denominator=[(tau) 1]
  Ω3 [rad/s] : Outport
  Ω3_dot : Outport  Port=2
  wires:
  Gain/1 -> Transfer Fcn/1
  Throttle3 [%]/1 -> Gain/1
  Transfer Fcn/1 -> Ω3_dot/1, Integrator/1
  Integrator/1 -> Bias/1
  Bias/1 -> Ω3 [rad/s]/1

== system TiltCopter_TOSTO_v3/TiltCopter/Actuators/ESC+Brushless4 ==
  Throttle4 [%] : Inport
  Bias : Bias  Bias=x1(2)
  Gain : Gain  Gain=x1(1)
  Integrator : Integrator
  Transfer Fcn : TransferFcn  Numerator=[-1 0]  Denominator=[(tau) 1]
  Ω4 [rad/s] : Outport
  "Ω4_dot " : Outport  Port=2
  wires:
  Gain/1 -> Transfer Fcn/1
  Throttle4 [%]/1 -> Gain/1
  Transfer Fcn/1 -> "Ω4_dot "/1, Integrator/1
  Integrator/1 -> Bias/1
  Bias/1 -> Ω4 [rad/s]/1

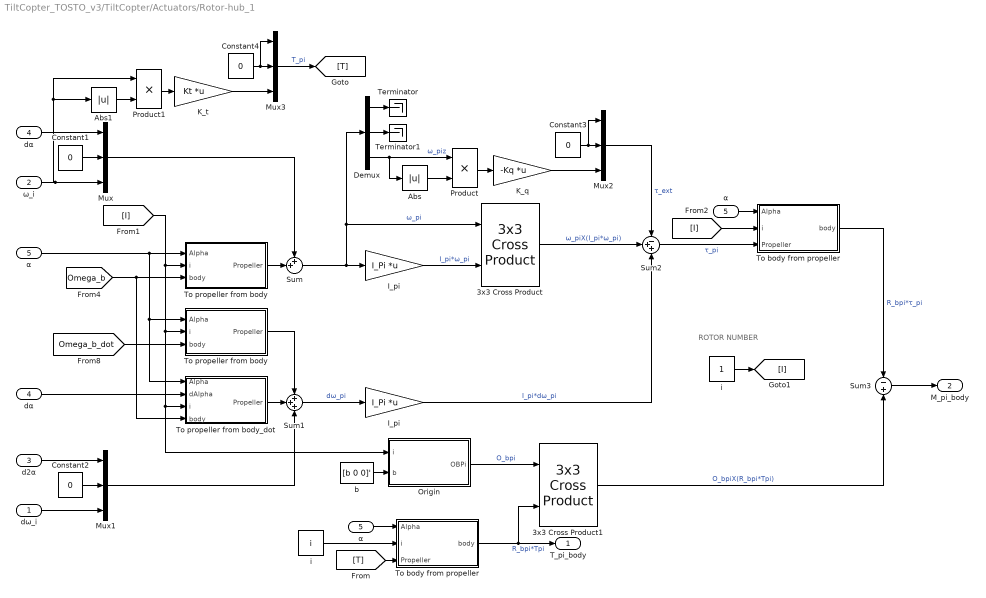
== system TiltCopter_TOSTO_v3/TiltCopter/Actuators/Rotor-hub_1 ==
  note: ROTOR NUMBER
  dω_i : Inport
  ω_i : Inport  Port=2
  d2α : Inport  Port=3
  dα : Inport  Port=4
  α : Inport  Port=5
  3x3 Cross Product : aerolibutil/3x3 Cross Product
  3x3 Cross Product1 : aerolibutil/3x3 Cross Product
  Abs : Abs
  Abs1 : Abs
  Constant{1..4} (4 alike) : Constant  Value=0
  Demux : Demux  Outputs=3
  I_pi : Gain  Gain=I_Pi  Multiplication=Matrix(K*u)
  "I_pi " : Gain  Gain=I_Pi  Multiplication=Matrix(K*u)
  K_q : Gain  Gain=-Kq  Multiplication=Matrix(K*u)
  K_t : Gain  Gain=Kt  Multiplication=Matrix(K*u)
  Mux{,1..3} (4 alike) : Mux  Inputs=3
  Origin : MATLAB Function  TreatAsAtomicUnit=on
  Product : Product
  Product1 : Product
  Sum : Sum  Inputs=++|
  Sum1 : Sum  Inputs=+++
  Sum2 : Sum  Inputs=-++
  Sum3 : Sum  Inputs=-|+
  Terminator : Terminator
  Terminator1 : Terminator
  To body from propeller : MATLAB Function  TreatAsAtomicUnit=on
  "To body from propeller " : MATLAB Function  TreatAsAtomicUnit=on
  To propeller from body : MATLAB Function  TreatAsAtomicUnit=on
  "To propeller from body " : MATLAB Function  TreatAsAtomicUnit=on
  To propeller from body_dot : MATLAB Function  TreatAsAtomicUnit=on
  b : Constant  Value=[b 0 0]'
  "dα " : InportShadow  Port=4
  i : Constant
  "i " : Constant  Value=i
  "α " : InportShadow  Port=5
  "α  " : InportShadow  Port=5
  " T_pi_body" : Outport
  " M_pi_body" : Outport  Port=2
  wires:
  α/1 -> To propeller from body/1(Alpha), "To propeller from body "/1(Alpha), To propeller from body_dot/1(Alpha)
  [Omega_b] -> To propeller from body/3(body), To propeller from body_dot/4(body)
  [I] -> Origin/1(i), To propeller from body_dot/3(i), "To propeller from body "/2(i), To propeller from body/2(i)
  Constant1/1 -> Mux/2
  Sum/1 -> Demux/1, 3x3 Cross Product/1, "I_pi "/1  "ω_pi"
  Constant2/1 -> Mux1/2
  [Omega_b_dot] -> "To propeller from body "/3(body)
  To propeller from body_dot/1(Propeller) -> Sum1/2
  Sum1/1 -> I_pi/1  "dω_pi"
  Mux1/1 -> Sum1/3
  To propeller from body/1(Propeller) -> Sum/2
  Mux/1 -> Sum/1
  "To propeller from body "/1(Propeller) -> Sum1/1
  "I_pi "/1 -> 3x3 Cross Product/2  "I_pi*ω_pi"
  3x3 Cross Product/1 -> Sum2/2  "ω_piX(I_pi*ω_pi)"
  I_pi/1 -> Sum2/3  "I_pi*dω_pi"
  Mux2/1 -> Sum2/1  "τ_ext"
  Constant3/1 -> Mux2/1, Mux2/2
  K_q/1 -> Mux2/3
  Demux/1 -> Terminator/1
  Demux/2 -> Terminator1/1
  Demux/3 -> Abs/1, Product/1  "ω_piz"
  Product/1 -> K_q/1
  Abs/1 -> Product/2
  Product1/1 -> K_t/1
  Abs1/1 -> Product1/2
  b/1 -> Origin/2(b)
  "α "/1 -> To body from propeller/1(Alpha)
  "i "/1 -> To body from propeller/2(i)
  "dα "/1 -> To propeller from body_dot/2(dAlpha)
  Origin/1(OBPi) -> 3x3 Cross Product1/1  "O_bpi"
  [T] -> To body from propeller/3(Propeller)
  To body from propeller/1(body) -> 3x3 Cross Product1/2, " T_pi_body"/1  "R_bpi*Tpi"
  3x3 Cross Product1/1 -> Sum3/2  "O_bpiX(R_bpi*Tpi)"
  "α  "/1 -> "To body from propeller "/1(Alpha)
  [I] -> "To body from propeller "/2(i)
  Sum2/1 -> "To body from propeller "/3(Propeller)  "τ_pi"
  "To body from propeller "/1(body) -> Sum3/1  "R_bpi*τ_pi"
  Sum3/1 -> " M_pi_body"/1
  i/1 -> [I]
  dα/1 -> Mux/1
  ω_i/1 -> Product1/1, Abs1/1, Mux/3
  Constant4/1 -> Mux3/1, Mux3/2
  Mux3/1 -> [T]  "T_pi"
  K_t/1 -> Mux3/3
  d2α/1 -> Mux1/1
  dω_i/1 -> Mux1/3

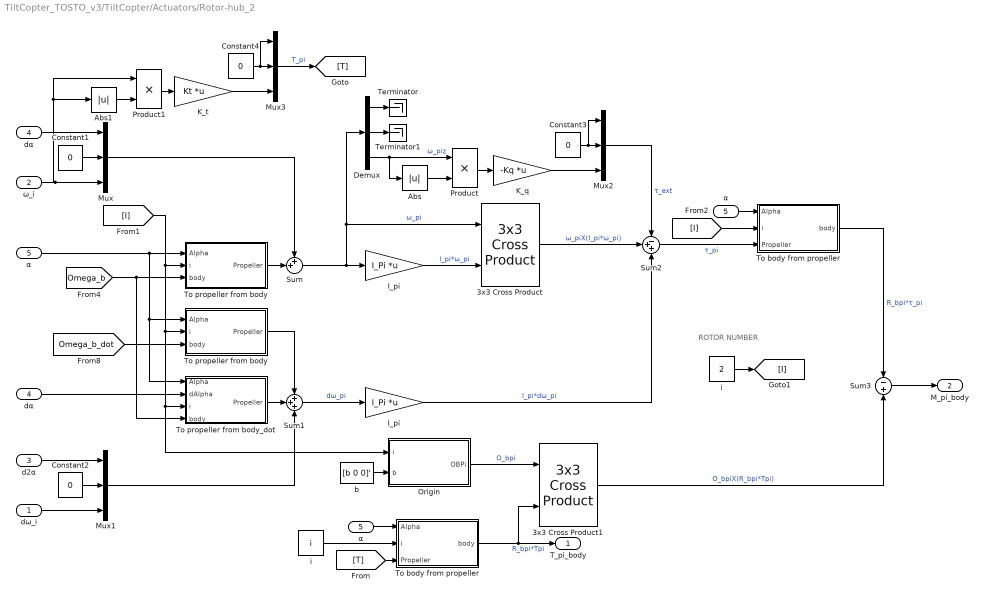
== system TiltCopter_TOSTO_v3/TiltCopter/Actuators/Rotor-hub_2 ==
  note: ROTOR NUMBER
  dω_i : Inport
  ω_i : Inport  Port=2
  d2α : Inport  Port=3
  dα : Inport  Port=4
  α : Inport  Port=5
  3x3 Cross Product : aerolibutil/3x3 Cross Product
  3x3 Cross Product1 : aerolibutil/3x3 Cross Product
  Abs : Abs
  Abs1 : Abs
  Constant{1..4} (4 alike) : Constant  Value=0
  Demux : Demux  Outputs=3
  I_pi : Gain  Gain=I_Pi  Multiplication=Matrix(K*u)
  "I_pi " : Gain  Gain=I_Pi  Multiplication=Matrix(K*u)
  K_q : Gain  Gain=-Kq  Multiplication=Matrix(K*u)
  K_t : Gain  Gain=Kt  Multiplication=Matrix(K*u)
  Mux{,1..3} (4 alike) : Mux  Inputs=3
  Origin : MATLAB Function  TreatAsAtomicUnit=on
  Product : Product
  Product1 : Product
  Sum : Sum  Inputs=++|
  Sum1 : Sum  Inputs=+++
  Sum2 : Sum  Inputs=-++
  Sum3 : Sum  Inputs=-|+
  Terminator : Terminator
  Terminator1 : Terminator
  To body from propeller : MATLAB Function  TreatAsAtomicUnit=on
  "To body from propeller " : MATLAB Function  TreatAsAtomicUnit=on
  To propeller from body : MATLAB Function  TreatAsAtomicUnit=on
  "To propeller from body " : MATLAB Function  TreatAsAtomicUnit=on
  To propeller from body_dot : MATLAB Function  TreatAsAtomicUnit=on
  b : Constant  Value=[b 0 0]'
  "dα " : InportShadow  Port=4
  i : Constant  Value=2
  "i " : Constant  Value=i
  "α " : InportShadow  Port=5
  "α  " : InportShadow  Port=5
  " T_pi_body" : Outport
  " M_pi_body" : Outport  Port=2
  wires:
  dω_i/1 -> Mux1/3
  d2α/1 -> Mux1/1
  K_t/1 -> Mux3/3
  Mux3/1 -> [T]  "T_pi"
  Constant4/1 -> Mux3/2, Mux3/1
  ω_i/1 -> Mux/3, Abs1/1, Product1/1
  dα/1 -> Mux/1
  i/1 -> [I]
  Sum3/1 -> " M_pi_body"/1
  "To body from propeller "/1(body) -> Sum3/1  "R_bpi*τ_pi"
  Sum2/1 -> "To body from propeller "/3(Propeller)  "τ_pi"
  [I] -> "To body from propeller "/2(i)
  "α  "/1 -> "To body from propeller "/1(Alpha)
  3x3 Cross Product1/1 -> Sum3/2  "O_bpiX(R_bpi*Tpi)"
  To body from propeller/1(body) -> " T_pi_body"/1, 3x3 Cross Product1/2  "R_bpi*Tpi"
  [T] -> To body from propeller/3(Propeller)
  Origin/1(OBPi) -> 3x3 Cross Product1/1  "O_bpi"
  "dα "/1 -> To propeller from body_dot/2(dAlpha)
  "i "/1 -> To body from propeller/2(i)
  "α "/1 -> To body from propeller/1(Alpha)
  b/1 -> Origin/2(b)
  Abs1/1 -> Product1/2
  Product1/1 -> K_t/1
  Abs/1 -> Product/2
  Product/1 -> K_q/1
  Demux/3 -> Product/1, Abs/1  "ω_piz"
  Demux/2 -> Terminator1/1
  Demux/1 -> Terminator/1
  K_q/1 -> Mux2/3
  Constant3/1 -> Mux2/2, Mux2/1
  Mux2/1 -> Sum2/1  "τ_ext"
  I_pi/1 -> Sum2/3  "I_pi*dω_pi"
  3x3 Cross Product/1 -> Sum2/2  "ω_piX(I_pi*ω_pi)"
  "I_pi "/1 -> 3x3 Cross Product/2  "I_pi*ω_pi"
  "To propeller from body "/1(Propeller) -> Sum1/1
  Mux/1 -> Sum/1
  To propeller from body/1(Propeller) -> Sum/2
  Mux1/1 -> Sum1/3
  Sum1/1 -> I_pi/1  "dω_pi"
  To propeller from body_dot/1(Propeller) -> Sum1/2
  [Omega_b_dot] -> "To propeller from body "/3(body)
  Constant2/1 -> Mux1/2
  Sum/1 -> "I_pi "/1, 3x3 Cross Product/1, Demux/1  "ω_pi"
  Constant1/1 -> Mux/2
  [I] -> To propeller from body/2(i), "To propeller from body "/2(i), To propeller from body_dot/3(i), Origin/1(i)
  [Omega_b] -> To propeller from body_dot/4(body), To propeller from body/3(body)
  α/1 -> To propeller from body_dot/1(Alpha), "To propeller from body "/1(Alpha), To propeller from body/1(Alpha)

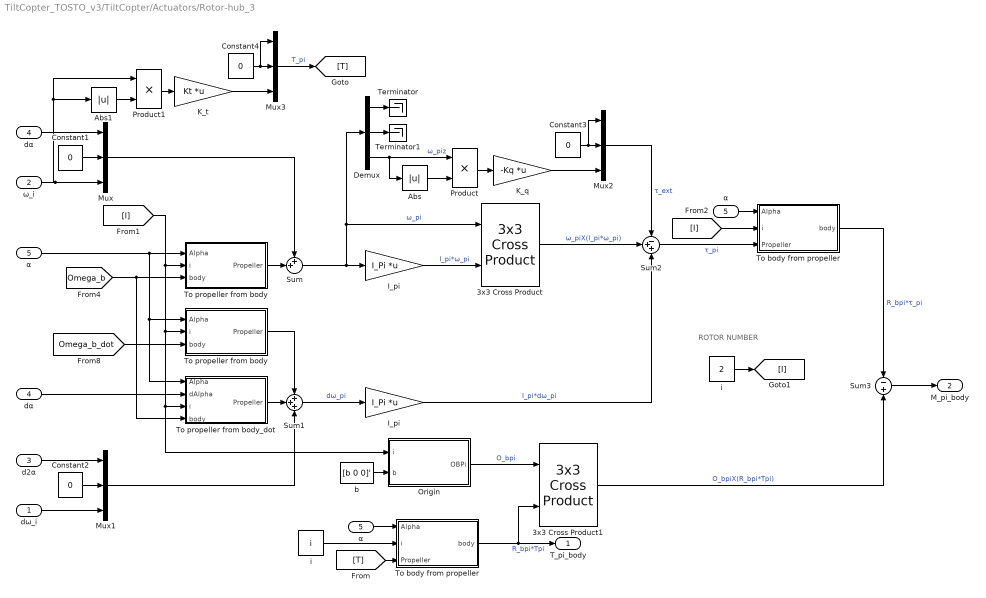
== system TiltCopter_TOSTO_v3/TiltCopter/Actuators/Rotor-hub_3 ==
  note: ROTOR NUMBER
  dω_i : Inport
  ω_i : Inport  Port=2
  d2α : Inport  Port=3
  dα : Inport  Port=4
  α : Inport  Port=5
  3x3 Cross Product : aerolibutil/3x3 Cross Product
  3x3 Cross Product1 : aerolibutil/3x3 Cross Product
  Abs : Abs
  Abs1 : Abs
  Constant{1..4} (4 alike) : Constant  Value=0
  Demux : Demux  Outputs=3
  I_pi : Gain  Gain=I_Pi  Multiplication=Matrix(K*u)
  "I_pi " : Gain  Gain=I_Pi  Multiplication=Matrix(K*u)
  K_q : Gain  Gain=-Kq  Multiplication=Matrix(K*u)
  K_t : Gain  Gain=Kt  Multiplication=Matrix(K*u)
  Mux{,1..3} (4 alike) : Mux  Inputs=3
  Origin : MATLAB Function  TreatAsAtomicUnit=on
  Product : Product
  Product1 : Product
  Sum : Sum  Inputs=++|
  Sum1 : Sum  Inputs=+++
  Sum2 : Sum  Inputs=-++
  Sum3 : Sum  Inputs=-|+
  Terminator : Terminator
  Terminator1 : Terminator
  To body from propeller : MATLAB Function  TreatAsAtomicUnit=on
  "To body from propeller " : MATLAB Function  TreatAsAtomicUnit=on
  To propeller from body : MATLAB Function  TreatAsAtomicUnit=on
  "To propeller from body " : MATLAB Function  TreatAsAtomicUnit=on
  To propeller from body_dot : MATLAB Function  TreatAsAtomicUnit=on
  b : Constant  Value=[b 0 0]'
  "dα " : InportShadow  Port=4
  i : Constant  Value=2
  "i " : Constant  Value=i
  "α " : InportShadow  Port=5
  "α  " : InportShadow  Port=5
  " T_pi_body" : Outport
  " M_pi_body" : Outport  Port=2
  wires:
  α/1 -> To propeller from body/1(Alpha), "To propeller from body "/1(Alpha), To propeller from body_dot/1(Alpha)
  [Omega_b] -> To propeller from body/3(body), To propeller from body_dot/4(body)
  [I] -> Origin/1(i), To propeller from body_dot/3(i), "To propeller from body "/2(i), To propeller from body/2(i)
  Constant1/1 -> Mux/2
  Sum/1 -> Demux/1, 3x3 Cross Product/1, "I_pi "/1  "ω_pi"
  Constant2/1 -> Mux1/2
  [Omega_b_dot] -> "To propeller from body "/3(body)
  To propeller from body_dot/1(Propeller) -> Sum1/2
  Sum1/1 -> I_pi/1  "dω_pi"
  Mux1/1 -> Sum1/3
  To propeller from body/1(Propeller) -> Sum/2
  Mux/1 -> Sum/1
  "To propeller from body "/1(Propeller) -> Sum1/1
  "I_pi "/1 -> 3x3 Cross Product/2  "I_pi*ω_pi"
  3x3 Cross Product/1 -> Sum2/2  "ω_piX(I_pi*ω_pi)"
  I_pi/1 -> Sum2/3  "I_pi*dω_pi"
  Mux2/1 -> Sum2/1  "τ_ext"
  Constant3/1 -> Mux2/1, Mux2/2
  K_q/1 -> Mux2/3
  Demux/1 -> Terminator/1
  Demux/2 -> Terminator1/1
  Demux/3 -> Abs/1, Product/1  "ω_piz"
  Product/1 -> K_q/1
  Abs/1 -> Product/2
  Product1/1 -> K_t/1
  Abs1/1 -> Product1/2
  b/1 -> Origin/2(b)
  "α "/1 -> To body from propeller/1(Alpha)
  "i "/1 -> To body from propeller/2(i)
  "dα "/1 -> To propeller from body_dot/2(dAlpha)
  Origin/1(OBPi) -> 3x3 Cross Product1/1  "O_bpi"
  [T] -> To body from propeller/3(Propeller)
  To body from propeller/1(body) -> 3x3 Cross Product1/2, " T_pi_body"/1  "R_bpi*Tpi"
  3x3 Cross Product1/1 -> Sum3/2  "O_bpiX(R_bpi*Tpi)"
  "α  "/1 -> "To body from propeller "/1(Alpha)
  [I] -> "To body from propeller "/2(i)
  Sum2/1 -> "To body from propeller "/3(Propeller)  "τ_pi"
  "To body from propeller "/1(body) -> Sum3/1  "R_bpi*τ_pi"
  Sum3/1 -> " M_pi_body"/1
  i/1 -> [I]
  dα/1 -> Mux/1
  ω_i/1 -> Product1/1, Abs1/1, Mux/3
  Constant4/1 -> Mux3/1, Mux3/2
  Mux3/1 -> [T]  "T_pi"
  K_t/1 -> Mux3/3
  d2α/1 -> Mux1/1
  dω_i/1 -> Mux1/3

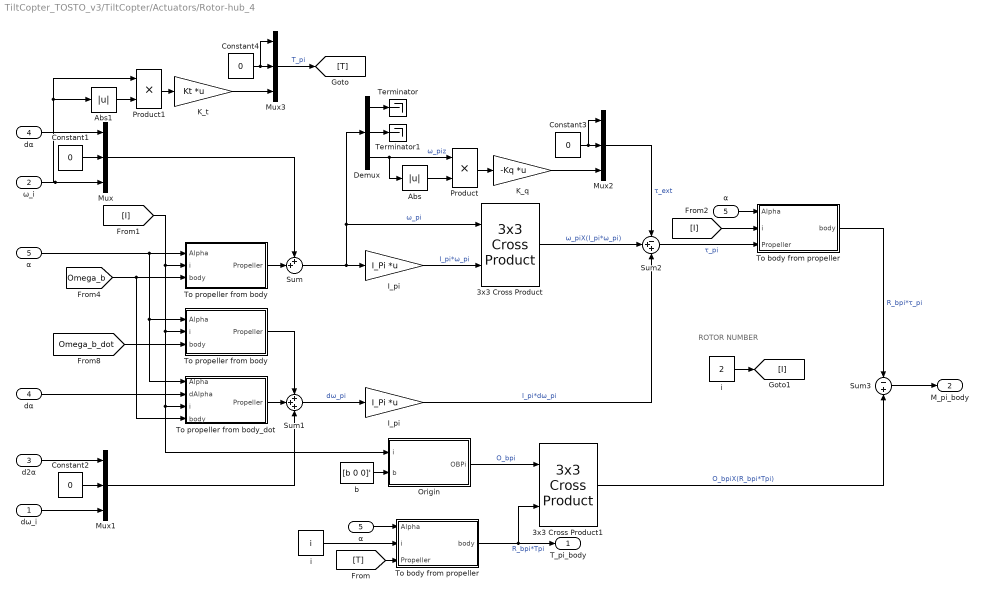
== system TiltCopter_TOSTO_v3/TiltCopter/Actuators/Rotor-hub_4 ==
  note: ROTOR NUMBER
  dω_i : Inport
  ω_i : Inport  Port=2
  d2α : Inport  Port=3
  dα : Inport  Port=4
  α : Inport  Port=5
  3x3 Cross Product : aerolibutil/3x3 Cross Product
  3x3 Cross Product1 : aerolibutil/3x3 Cross Product
  Abs : Abs
  Abs1 : Abs
  Constant{1..4} (4 alike) : Constant  Value=0
  Demux : Demux  Outputs=3
  I_pi : Gain  Gain=I_Pi  Multiplication=Matrix(K*u)
  "I_pi " : Gain  Gain=I_Pi  Multiplication=Matrix(K*u)
  K_q : Gain  Gain=-Kq  Multiplication=Matrix(K*u)
  K_t : Gain  Gain=Kt  Multiplication=Matrix(K*u)
  Mux{,1..3} (4 alike) : Mux  Inputs=3
  Origin : MATLAB Function  TreatAsAtomicUnit=on
  Product : Product
  Product1 : Product
  Sum : Sum  Inputs=++|
  Sum1 : Sum  Inputs=+++
  Sum2 : Sum  Inputs=-++
  Sum3 : Sum  Inputs=-|+
  Terminator : Terminator
  Terminator1 : Terminator
  To body from propeller : MATLAB Function  TreatAsAtomicUnit=on
  "To body from propeller " : MATLAB Function  TreatAsAtomicUnit=on
  To propeller from body : MATLAB Function  TreatAsAtomicUnit=on
  "To propeller from body " : MATLAB Function  TreatAsAtomicUnit=on
  To propeller from body_dot : MATLAB Function  TreatAsAtomicUnit=on
  b : Constant  Value=[b 0 0]'
  "dα " : InportShadow  Port=4
  i : Constant  Value=2
  "i " : Constant  Value=i
  "α " : InportShadow  Port=5
  "α  " : InportShadow  Port=5
  " T_pi_body" : Outport
  " M_pi_body" : Outport  Port=2
  wires:
  dω_i/1 -> Mux1/3
  d2α/1 -> Mux1/1
  K_t/1 -> Mux3/3
  Mux3/1 -> [T]  "T_pi"
  Constant4/1 -> Mux3/2, Mux3/1
  ω_i/1 -> Mux/3, Abs1/1, Product1/1
  dα/1 -> Mux/1
  i/1 -> [I]
  Sum3/1 -> " M_pi_body"/1
  "To body from propeller "/1(body) -> Sum3/1  "R_bpi*τ_pi"
  Sum2/1 -> "To body from propeller "/3(Propeller)  "τ_pi"
  [I] -> "To body from propeller "/2(i)
  "α  "/1 -> "To body from propeller "/1(Alpha)
  3x3 Cross Product1/1 -> Sum3/2  "O_bpiX(R_bpi*Tpi)"
  To body from propeller/1(body) -> " T_pi_body"/1, 3x3 Cross Product1/2  "R_bpi*Tpi"
  [T] -> To body from propeller/3(Propeller)
  Origin/1(OBPi) -> 3x3 Cross Product1/1  "O_bpi"
  "dα "/1 -> To propeller from body_dot/2(dAlpha)
  "i "/1 -> To body from propeller/2(i)
  "α "/1 -> To body from propeller/1(Alpha)
  b/1 -> Origin/2(b)
  Abs1/1 -> Product1/2
  Product1/1 -> K_t/1
  Abs/1 -> Product/2
  Product/1 -> K_q/1
  Demux/3 -> Product/1, Abs/1  "ω_piz"
  Demux/2 -> Terminator1/1
  Demux/1 -> Terminator/1
  K_q/1 -> Mux2/3
  Constant3/1 -> Mux2/2, Mux2/1
  Mux2/1 -> Sum2/1  "τ_ext"
  I_pi/1 -> Sum2/3  "I_pi*dω_pi"
  3x3 Cross Product/1 -> Sum2/2  "ω_piX(I_pi*ω_pi)"
  "I_pi "/1 -> 3x3 Cross Product/2  "I_pi*ω_pi"
  "To propeller from body "/1(Propeller) -> Sum1/1
  Mux/1 -> Sum/1
  To propeller from body/1(Propeller) -> Sum/2
  Mux1/1 -> Sum1/3
  Sum1/1 -> I_pi/1  "dω_pi"
  To propeller from body_dot/1(Propeller) -> Sum1/2
  [Omega_b_dot] -> "To propeller from body "/3(body)
  Constant2/1 -> Mux1/2
  Sum/1 -> "I_pi "/1, 3x3 Cross Product/1, Demux/1  "ω_pi"
  Constant1/1 -> Mux/2
  [I] -> To propeller from body/2(i), "To propeller from body "/2(i), To propeller from body_dot/3(i), Origin/1(i)
  [Omega_b] -> To propeller from body_dot/4(body), To propeller from body/3(body)
  α/1 -> To propeller from body_dot/1(Alpha), "To propeller from body "/1(Alpha), To propeller from body/1(Alpha)

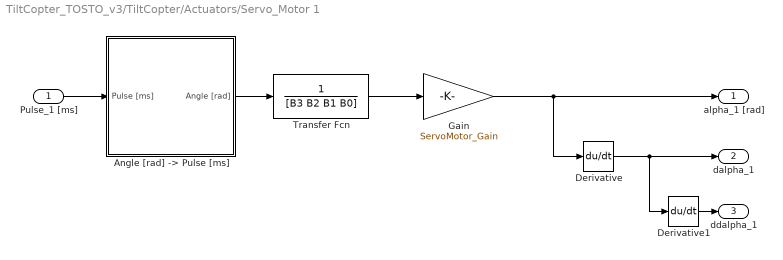
== system TiltCopter_TOSTO_v3/TiltCopter/Actuators/Servo_Motor 1 ==
  Pulse_1 [ms] : Inport
  "Angle [rad] -> Pulse [ms]" : Subsystem
  Derivative : Derivative
  Derivative1 : Derivative
  Gain : Gain  Gain=ServoMotor_Gain
  Transfer Fcn : TransferFcn  Denominator=[B3 B2 B1 B0]
  alpha_1 [rad] : Outport
  dalpha_1 : Outport  Port=2
  ddalpha_1 : Outport  Port=3
  wires:
  Gain/1 -> Derivative/1, alpha_1 [rad]/1
  Transfer Fcn/1 -> Gain/1
  "Angle [rad] -> Pulse [ms]"/1(Angle [rad]) -> Transfer Fcn/1
  Pulse_1 [ms]/1 -> "Angle [rad] -> Pulse [ms]"/1(Pulse [ms])
  Derivative/1 -> dalpha_1/1, Derivative1/1
  Derivative1/1 -> ddalpha_1/1

== system TiltCopter_TOSTO_v3/TiltCopter/Actuators/Servo_Motor 2 ==
  Pulse_2 [ms] : Inport
  "Angle [rad] -> Pulse [ms]" : Subsystem
  Derivative : Derivative
  Derivative1 : Derivative
  Gain : Gain  Gain=ServoMotor_Gain
  Transfer Fcn : TransferFcn  Denominator=[B3 B2 B1 B0]
  alpha_2 [rad] : Outport
  dalpha_2 : Outport  Port=2
  ddalpha_2 : Outport  Port=3
  wires:
  Gain/1 -> Derivative/1, alpha_2 [rad]/1
  Transfer Fcn/1 -> Gain/1
  "Angle [rad] -> Pulse [ms]"/1(Angle [rad]) -> Transfer Fcn/1
  Pulse_2 [ms]/1 -> "Angle [rad] -> Pulse [ms]"/1(Pulse [ms])
  Derivative/1 -> dalpha_2/1, Derivative1/1
  Derivative1/1 -> ddalpha_2/1

== system TiltCopter_TOSTO_v3/TiltCopter/Actuators/Servo_Motor 3 ==
  Pulse_3 [ms] : Inport
  "Angle [rad] -> Pulse [ms]" : Subsystem
  Derivative : Derivative
  Derivative1 : Derivative
  Gain : Gain  Gain=ServoMotor_Gain
  Transfer Fcn : TransferFcn  Denominator=[B3 B2 B1 B0]
  alpha_3 [rad] : Outport
  dalpha_3 : Outport  Port=2
  ddalpha_3 : Outport  Port=3
  wires:
  Gain/1 -> Derivative/1, alpha_3 [rad]/1
  Transfer Fcn/1 -> Gain/1
  "Angle [rad] -> Pulse [ms]"/1(Angle [rad]) -> Transfer Fcn/1
  Pulse_3 [ms]/1 -> "Angle [rad] -> Pulse [ms]"/1(Pulse [ms])
  Derivative/1 -> dalpha_3/1, Derivative1/1
  Derivative1/1 -> ddalpha_3/1

== system TiltCopter_TOSTO_v3/TiltCopter/Actuators/Servo_Motor 4 ==
  Pulse_4 [ms] : Inport
  "Angle [rad] -> Pulse [ms]" : Subsystem
  Derivative : Derivative
  Derivative1 : Derivative
  Gain : Gain  Gain=ServoMotor_Gain
  Transfer Fcn : TransferFcn  Denominator=[B3 B2 B1 B0]
  alpha_4 [rad] : Outport
  dalpha_4 : Outport  Port=2
  ddalpha_4 : Outport  Port=3
  wires:
  Gain/1 -> Derivative/1, alpha_4 [rad]/1
  Transfer Fcn/1 -> Gain/1
  "Angle [rad] -> Pulse [ms]"/1(Angle [rad]) -> Transfer Fcn/1
  Pulse_4 [ms]/1 -> "Angle [rad] -> Pulse [ms]"/1(Pulse [ms])
  Derivative1/1 -> ddalpha_4/1
  Derivative/1 -> Derivative1/1, dalpha_4/1

== system TiltCopter_TOSTO_v3/TiltCopter/Actuators/Traslational Force_1 ==
  alpha_i : Inport
  omega_i : Inport  Port=2
  Product : Product  Multiplication=Matrix(*)
  R_BP1 : MATLAB Function  TreatAsAtomicUnit=on
  Thrust computation : Subsystem
  F_i : Outport
  wires:
  Thrust computation/1(Vector_Thrust_i) -> Product/2
  Product/1 -> F_i/1
  omega_i/1 -> Thrust computation/1(omega_i)
  R_BP1/1(Rotation_matrix) -> Product/1
  alpha_i/1 -> R_BP1/1(alpha_1)

== system TiltCopter_TOSTO_v3/TiltCopter/Actuators/Traslational Force_2 ==
  alpha_i : Inport
  omega_i : Inport  Port=2
  Product : Product  Multiplication=Matrix(*)
  R_BP2 : MATLAB Function  TreatAsAtomicUnit=on
  Thrust computation : Subsystem
  F_i : Outport
  wires:
  Thrust computation/1(Vector_Thrust_i) -> Product/2
  Product/1 -> F_i/1
  omega_i/1 -> Thrust computation/1(omega_i)
  R_BP2/1(Rotation_matrix) -> Product/1
  alpha_i/1 -> R_BP2/1(alpha_2)

== system TiltCopter_TOSTO_v3/TiltCopter/Actuators/Traslational Force_3 ==
  alpha_i : Inport
  omega_i : Inport  Port=2
  Product : Product  Multiplication=Matrix(*)
  R_BP3 : MATLAB Function  TreatAsAtomicUnit=on
  Thrust computation : Subsystem
  F_i : Outport
  wires:
  Thrust computation/1(Vector_Thrust_i) -> Product/2
  Product/1 -> F_i/1
  omega_i/1 -> Thrust computation/1(omega_i)
  R_BP3/1(Rotation_matrix) -> Product/1
  alpha_i/1 -> R_BP3/1(alpha_3)
